simulink model "SR25"  (R2024a)
settings: Solver=FixedStepDiscrete  StartTime=0.0  StopTime=5  FixedStep=0.01  RelTol=1e-3  EnableMultiTasking=on
PreLoadFcn:
  | try, model_open; catch, disp('Error occurred while executing model pre-load callback: model_open.m'); disp('Please assure that the MATLAB working directory is set to the model directory before opening.'); end
InitFcn:
  | try, model_open; catch, end
undefined symbols (not defined in the file or in its folder): dt, GCM, raptor_get_safe_string, raptor_xcp_function
libraries: Raptor_lib x40, Utilities x13, TireTemperature x12, simulink x5, IO x5, APPS_BSPC x4, RotorTemperature x4, FlowRate x3, Cooling x2, BMS x2, Brakes x2, StateMachine x2
(part 2 of 3)

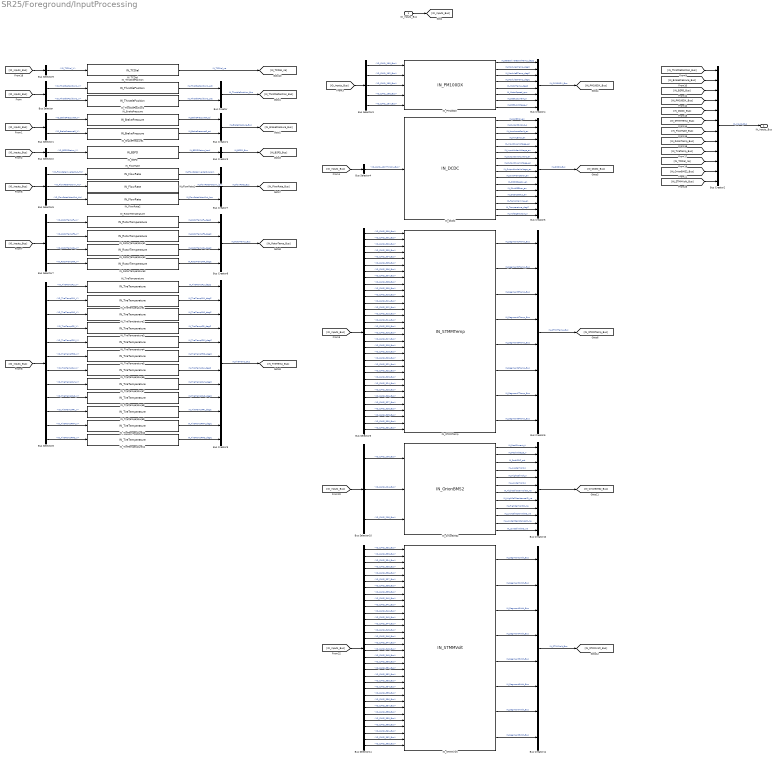
== system SR25/Foreground/InputProcessing ==
  IO_Inputs_Bus : Inport
  Bus Creator : BusCreator  Inputs=2
  Bus Creator1 : BusCreator  Inputs=2
  Bus Creator10 : BusCreator  Inputs=12
  Bus Creator11 : BusCreator  Inputs=8
  Bus Creator2 : BusCreator  Inputs=12
  Bus Creator3 : BusCreator  Inputs=1
  Bus Creator4 : BusCreator  Inputs=8
  Bus Creator5 : BusCreator  Inputs=16
  Bus Creator6 : BusCreator  Inputs=8
  Bus Creator7 : BusCreator  Inputs=3
  Bus Creator8 : BusCreator  Inputs=4
  Bus Creator9 : BusCreator  Inputs=12
  Bus Selector : BusSelector  OutputSignals=IO_AnalogInputs_Bus.IO_ThrottlePosition1_V,IO_AnalogInputs_Bus.IO_ThrottlePosition2_V
  Bus Selector1 : BusSelector  OutputSignals=IO_AnalogInputs_Bus.IO_BrakePressureF_V,IO_AnalogInputs_Bus.IO_BrakePressureR_V
  Bus Selector10 : BusSelector  OutputSignals=IO_CANInputs_Bus.IO_CAN2_Bus.IO_CAN2_BMS_Bus.IO_CAN2_200_Bus,IO_CANInputs_Bus.IO_CAN2_Bus.IO_CAN2_BMS_Bus.IO_CAN2_204_Bus,IO_CANInputs_Bus.IO_CAN2_Bus.IO_CAN2_BMS_Bus.IO_CAN2_208_Bus
  Bus Selector11 : BusSelector  OutputSignals=IO_CANInputs_Bus.IO_CAN2_Bus.IO_CAN2_STMM_Bus.IO_CAN2_STMM_Volt_Bus.IO_CAN2_332_Bus,IO_CANInputs_Bus.IO_CAN2_Bus.IO_CAN2_STMM_Bus.IO_CAN2_STMM_Volt_Bus.IO_CAN2_333_Bus,IO_CANInputs_Bus.IO_CAN2_Bus.IO_CAN2_STMM_Bus.IO_CAN2_STMM_Volt_Bus.IO_CAN2_334_Bus,IO_CANInputs_Bus.IO_CAN2_Bus.IO_CAN2_STMM_Bus.IO_CAN2_STMM_Volt_Bus.IO_CAN2_335_Bus,IO_CANInputs_Bus.IO_CAN2_Bus.IO_CAN2_STMM_Bus.IO_CAN2_STMM_Volt_Bus.IO_CAN2_336_Bus,IO_CANInputs_Bus.IO_CAN2_Bus.IO_CAN2_STMM_Bus.IO_CAN2_STMM_Volt_Bus.IO_CAN2_337_Bus,IO_CANInputs_Bus.IO_CAN2_Bus.IO_CAN2_STMM_Bus.IO_CAN2_STMM_Volt_Bus.IO_CAN2_338_Bus,IO_CANInputs_Bus.IO_CAN2_Bus.IO_CAN2_STMM_Bus.IO_CAN2_STMM_Volt_Bus.IO_CAN2_339_Bus,IO_CANInputs_Bus.IO_CAN2_Bus.IO_CAN2_STMM_Bus.IO_CAN2_STMM_Volt_Bus.IO_CAN2_340_Bus,IO_CANInputs_Bus.IO_CAN2_Bus.IO_CAN2_STMM_Bus.IO_CAN2_STMM_Volt_Bus.IO_CAN2_341_Bus,IO_CANInputs_Bus.IO_CAN2_Bus.IO_CAN2_STMM_Bus.IO_CAN2_STMM_Volt_Bus.IO_CAN2_342_Bus,IO_CANInputs_Bus.IO_CAN2_Bus.IO_CAN2_STMM_Bus.IO_CAN2_STMM_Volt_Bus.IO_CAN2_343_Bus,IO_CANInputs_Bus.IO_CAN2_Bus.IO_CAN2_STMM_Bus.IO_CAN2_STMM_Volt_Bus.IO_CAN2_344_Bus,IO_CANInputs_Bus.IO_CAN2_Bus.IO_CAN2_STMM_Bus.IO_CAN2_STMM_Volt_Bus.IO_CAN2_345_Bus,IO_CANInputs_Bus.IO_CAN2_Bus.IO_CAN2_STMM_Bus.IO_CAN2_STMM_Volt_Bus.IO_CAN2_346_Bus,IO_CANInputs_Bus.IO_CAN2_Bus.IO_CAN2_STMM_Bus.IO_CAN2_STMM_Volt_Bus.IO_CAN2_347_Bus,IO_CANInputs_Bus.IO_CAN2_Bus.IO_CAN2_STMM_Bus.IO_CAN2_STMM_Volt_Bus.IO_CAN2_348_Bus,IO_CANInputs_Bus.IO_CAN2_Bus.IO_CAN2_STMM_Bus.IO_CAN2_STMM_Volt_Bus.IO_CAN2_349_Bus,IO_CANInputs_Bus.IO_CAN2_Bus.IO_CAN2_STMM_Bus.IO_CAN2_STMM_Volt_Bus.IO_CAN2_350_Bus,IO_CANInputs_Bus.IO_CAN2_Bus.IO_CAN2_STMM_Bus.IO_CAN2_STMM_Volt_Bus.IO_CAN2_351_Bus,IO_CANInputs_Bus.IO_CAN2_Bus.IO_CAN2_STMM_Bus.IO_CAN2_STMM_Volt_Bus.IO_CAN2_352_Bus,IO_CANInputs_Bus.IO_CAN2_Bus.IO_CAN2_STMM_Bus.IO_CAN2_STMM_Volt_Bus.IO_CAN2_353_Bus,IO_CANInputs_Bus.IO_CAN2_Bus.IO_CAN2_STMM_Bus.IO_CAN2_STMM_Volt_Bus.IO_CAN2_354_Bus,IO_CANInputs_Bus.IO_CAN2_Bus.IO_CAN2_STMM_Bus.IO_CAN2_STMM_Volt_Bus.IO_CAN2_355_Bus,IO_CANInputs_Bus.IO_CAN2_Bus.IO_CAN2_STMM_Bus.IO_CAN2_STMM_Volt_Bus.IO_CAN2_356_Bus,IO_CANInputs_Bus.IO_CAN2_Bus.IO_CAN2_STMM_Bus.IO_CAN2_STMM_Volt_Bus.IO_CAN2_357_Bus,IO_CANInputs_Bus.IO_CAN2_Bus.IO_CAN2_STMM_Bus.IO_CAN2_STMM_Volt_Bus.IO_CAN2_358_Bus,IO_CANInputs_Bus.IO_CAN2_Bus.IO_CAN2_STMM_Bus.IO_CAN2_STMM_Volt_Bus.IO_CAN2_359_Bus,IO_CANInputs_Bus.IO_CAN2_Bus.IO_CAN2_STMM_Bus.IO_CAN2_STMM_Volt_Bus.IO_CAN2_360_Bus,IO_CANInputs_Bus.IO_CAN2_Bus.IO_CAN2_STMM_Bus.IO_CAN2_STMM_Volt_Bus.IO_CAN2_361_Bus,IO_CANInputs_Bus.IO_CAN2_Bus.IO_CAN2_STMM_Bus.IO_CAN2_STMM_Volt_Bus.IO_CAN2_362_Bus,IO_CANInputs_Bus.IO_CAN2_Bus.IO_CAN2_STMM_Bus.IO_CAN2_STMM_Volt_Bus.IO_CAN2_363_Bus
  Bus Selector2 : BusSelector  OutputSignals=IO_AnalogInputs_Bus.IO_BSPDStatus_V
  Bus Selector3 : BusSelector  OutputSignals=IO_CANInputs_Bus.IO_CAN1_Bus.IO_CAN1_PM100DX_Bus.IO_CAN1_160_Bus,IO_CANInputs_Bus.IO_CAN1_Bus.IO_CAN1_PM100DX_Bus.IO_CAN1_162_Bus,IO_CANInputs_Bus.IO_CAN1_Bus.IO_CAN1_PM100DX_Bus.IO_CAN1_165_Bus,IO_CANInputs_Bus.IO_CAN1_Bus.IO_CAN1_PM100DX_Bus.IO_CAN1_166_Bus,IO_CANInputs_Bus.IO_CAN1_Bus.IO_CAN1_PM100DX_Bus.IO_CAN1_167_Bus
  Bus Selector4 : BusSelector  OutputSignals=IO_CANInputs_Bus.IO_CAN1_Bus.IO_CAN1_DCDC_Bus.IO_CAN1_402772111_Bus
  Bus Selector5 : BusSelector  OutputSignals=IO_CANInputs_Bus.IO_CAN2_Bus.IO_CAN2_STMM_Bus.IO_CAN2_STMM_Temp_Bus.IO_CAN2_300_Bus,IO_CANInputs_Bus.IO_CAN2_Bus.IO_CAN2_STMM_Bus.IO_CAN2_STMM_Temp_Bus.IO_CAN2_301_Bus,IO_CANInputs_Bus.IO_CAN2_Bus.IO_CAN2_STMM_Bus.IO_CAN2_STMM_Temp_Bus.IO_CAN2_302_Bus,IO_CANInputs_Bus.IO_CAN2_Bus.IO_CAN2_STMM_Bus.IO_CAN2_STMM_Temp_Bus.IO_CAN2_303_Bus,IO_CANInputs_Bus.IO_CAN2_Bus.IO_CAN2_STMM_Bus.IO_CAN2_STMM_Temp_Bus.IO_CAN2_304_Bus,IO_CANInputs_Bus.IO_CAN2_Bus.IO_CAN2_STMM_Bus.IO_CAN2_STMM_Temp_Bus.IO_CAN2_305_Bus,IO_CANInputs_Bus.IO_CAN2_Bus.IO_CAN2_STMM_Bus.IO_CAN2_STMM_Temp_Bus.IO_CAN2_306_Bus,IO_CANInputs_Bus.IO_CAN2_Bus.IO_CAN2_STMM_Bus.IO_CAN2_STMM_Temp_Bus.IO_CAN2_307_Bus,IO_CANInputs_Bus.IO_CAN2_Bus.IO_CAN2_STMM_Bus.IO_CAN2_STMM_Temp_Bus.IO_CAN2_308_Bus,IO_CANInputs_Bus.IO_CAN2_Bus.IO_CAN2_STMM_Bus.IO_CAN2_STMM_Temp_Bus.IO_CAN2_309_Bus,IO_CANInputs_Bus.IO_CAN2_Bus.IO_CAN2_STMM_Bus.IO_CAN2_STMM_Temp_Bus.IO_CAN2_310_Bus,IO_CANInputs_Bus.IO_CAN2_Bus.IO_CAN2_STMM_Bus.IO_CAN2_STMM_Temp_Bus.IO_CAN2_311_Bus,IO_CANInputs_Bus.IO_CAN2_Bus.IO_CAN2_STMM_Bus.IO_CAN2_STMM_Temp_Bus.IO_CAN2_312_Bus,IO_CANInputs_Bus.IO_CAN2_Bus.IO_CAN2_STMM_Bus.IO_CAN2_STMM_Temp_Bus.IO_CAN2_313_Bus,IO_CANInputs_Bus.IO_CAN2_Bus.IO_CAN2_STMM_Bus.IO_CAN2_STMM_Temp_Bus.IO_CAN2_314_Bus,IO_CANInputs_Bus.IO_CAN2_Bus.IO_CAN2_STMM_Bus.IO_CAN2_STMM_Temp_Bus.IO_CAN2_315_Bus,IO_CANInputs_Bus.IO_CAN2_Bus.IO_CAN2_STMM_Bus.IO_CAN2_STMM_Temp_Bus.IO_CAN2_316_Bus,IO_CANInputs_Bus.IO_CAN2_Bus.IO_CAN2_STMM_Bus.IO_CAN2_STMM_Temp_Bus.IO_CAN2_317_Bus,IO_CANInputs_Bus.IO_CAN2_Bus.IO_CAN2_STMM_Bus.IO_CAN2_STMM_Temp_Bus.IO_CAN2_318_Bus,IO_CANInputs_Bus.IO_CAN2_Bus.IO_CAN2_STMM_Bus.IO_CAN2_STMM_Temp_Bus.IO_CAN2_319_Bus,IO_CANInputs_Bus.IO_CAN2_Bus.IO_CAN2_STMM_Bus.IO_CAN2_STMM_Temp_Bus.IO_CAN2_320_Bus,IO_CANInputs_Bus.IO_CAN2_Bus.IO_CAN2_STMM_Bus.IO_CAN2_STMM_Temp_Bus.IO_CAN2_321_Bus,IO_CANInputs_Bus.IO_CAN2_Bus.IO_CAN2_STMM_Bus.IO_CAN2_STMM_Temp_Bus.IO_CAN2_322_Bus,IO_CANInputs_Bus.IO_CAN2_Bus.IO_CAN2_STMM_Bus.IO_CAN2_STMM_Temp_Bus.IO_CAN2_323_Bus,IO_CANInputs_Bus.IO_CAN2_Bus.IO_CAN2_STMM_Bus.IO_CAN2_STMM_Temp_Bus.IO_CAN2_324_Bus,IO_CANInputs_Bus.IO_CAN2_Bus.IO_CAN2_STMM_Bus.IO_CAN2_STMM_Temp_Bus.IO_CAN2_325_Bus,IO_CANInputs_Bus.IO_CAN2_Bus.IO_CAN2_STMM_Bus.IO_CAN2_STMM_Temp_Bus.IO_CAN2_326_Bus,IO_CANInputs_Bus.IO_CAN2_Bus.IO_CAN2_STMM_Bus.IO_CAN2_STMM_Temp_Bus.IO_CAN2_327_Bus,IO_CANInputs_Bus.IO_CAN2_Bus.IO_CAN2_STMM_Bus.IO_CAN2_STMM_Temp_Bus.IO_CAN2_328_Bus,IO_CANInputs_Bus.IO_CAN2_Bus.IO_CAN2_STMM_Bus.IO_CAN2_STMM_Temp_Bus.IO_CAN2_329_Bus,IO_CANInputs_Bus.IO_CAN2_Bus.IO_CAN2_STMM_Bus.IO_CAN2_STMM_Temp_Bus.IO_CAN2_330_Bus,IO_CANInputs_Bus.IO_CAN2_Bus.IO_CAN2_STMM_Bus.IO_CAN2_STMM_Temp_Bus.IO_CAN2_331_Bus
  Bus Selector6 : BusSelector  OutputSignals=IO_DigitalInputs_Bus.IO_FlowRateInverterOut_Hz,IO_DigitalInputs_Bus.IO_FlowRateMotorIn_Hz,IO_DigitalInputs_Bus.IO_FlowRateMotorOut_Hz
  Bus Selector7 : BusSelector  OutputSignals=IO_AnalogInputs_Bus.IO_RotorTempFL_V,IO_AnalogInputs_Bus.IO_RotorTempFR_V,IO_AnalogInputs_Bus.IO_RotorTempRL_V,IO_AnalogInputs_Bus.IO_RotorTempRR_V
  Bus Selector8 : BusSelector  OutputSignals=IO_AnalogInputs_Bus.IO_TireTempFLI_V,IO_AnalogInputs_Bus.IO_TireTempFLM_V,IO_AnalogInputs_Bus.IO_TireTempFLO_V,IO_AnalogInputs_Bus.IO_TireTempFRI_V,IO_AnalogInputs_Bus.IO_TireTempFRM_V,IO_AnalogInputs_Bus.IO_TireTempFRO_V,IO_AnalogInputs_Bus.IO_TireTempRLI_V,IO_AnalogInputs_Bus.IO_TireTempRLM_V,IO_AnalogInputs_Bus.IO_TireTempRLO_V,IO_AnalogInputs_Bus.IO_TireTempRRI_V,IO_AnalogInputs_Bus.IO_TireTempRRM_V,IO_AnalogInputs_Bus.IO_TireTempRRO_V
  Bus Selector9 : BusSelector  OutputSignals=IO_AnalogInputs_Bus.IO_TCDial_V
  IN_BSPD : BSPD/IN_BSPD  pos='Status'
  IN_BrakePressure : BrakePressure/IN_BrakePressure  pos='F'
  IN_BrakePressure1 : BrakePressure/IN_BrakePressure  pos='R'
  IN_DCDC : DCDC/IN_DCDC  SystemSampleTime=-1  VariantActivationTime=update diagram  AllowFlexibleInterface=on  Latency=0  AutoFrameSizeCalculation=off
  IN_FlowRate : FlowRate/IN_FlowRate  pos='InverterOut'
  IN_FlowRate1 : FlowRate/IN_FlowRate  pos='MotorIn'
  IN_FlowRate2 : FlowRate/IN_FlowRate  pos='MotorOut'
  IN_OrionBMS2 : OrionBMS2/IN_OrionBMS2  SystemSampleTime=-1  VariantActivationTime=update diagram  AllowFlexibleInterface=on  Latency=0  AutoFrameSizeCalculation=off
  IN_PM100DX : PM100DX/IN_PM100DX  SystemSampleTime=-1  VariantActivationTime=update diagram  AllowFlexibleInterface=on  Latency=0  AutoFrameSizeCalculation=off
  IN_RotorTemperature : RotorTemperature/IN_RotorTemperature  pos='FL'
  IN_RotorTemperature1 : RotorTemperature/IN_RotorTemperature  pos='FR'
  IN_RotorTemperature2 : RotorTemperature/IN_RotorTemperature  pos='RL'
  IN_RotorTemperature3 : RotorTemperature/IN_RotorTemperature  pos='RR'
  IN_STMMTemp : STMM/IN_STMMTemp  SystemSampleTime=-1  VariantActivationTime=update diagram  AllowFlexibleInterface=on  Latency=0  AutoFrameSizeCalculation=off
  IN_STMMVolt : STMM/IN_STMMVolt  SystemSampleTime=-1  VariantActivationTime=update diagram  AllowFlexibleInterface=on  Latency=0  AutoFrameSizeCalculation=off
  IN_TCDial : TCDial/IN_TCDial  pos=''
  IN_ThrottlePosition : ThrottlePosition/IN_ThrottlePosition  pos='1'
  IN_ThrottlePosition1 : ThrottlePosition/IN_ThrottlePosition  pos='2'
  IN_TireTemperature : TireTemperature/IN_TireTemperature  pos='FLI'
  IN_TireTemperature1 : TireTemperature/IN_TireTemperature  pos='FLM'
  IN_TireTemperature10 : TireTemperature/IN_TireTemperature  pos='RRM'
  IN_TireTemperature11 : TireTemperature/IN_TireTemperature  pos='RRO'
  IN_TireTemperature2 : TireTemperature/IN_TireTemperature  pos='FLO'
  IN_TireTemperature3 : TireTemperature/IN_TireTemperature  pos='FRI'
  IN_TireTemperature4 : TireTemperature/IN_TireTemperature  pos='FRM'
  IN_TireTemperature5 : TireTemperature/IN_TireTemperature  pos='FRO'
  IN_TireTemperature6 : TireTemperature/IN_TireTemperature  pos='RLI'
  IN_TireTemperature7 : TireTemperature/IN_TireTemperature  pos='RLM'
  IN_TireTemperature8 : TireTemperature/IN_TireTemperature  pos='RLO'
  IN_TireTemperature9 : TireTemperature/IN_TireTemperature  pos='RRI'
  IN_Inputs_Bus : Outport
  wires:
  Bus Selector/1 -> IN_ThrottlePosition/1  "<IO_ThrottlePosition1_V>"
  Bus Selector/2 -> IN_ThrottlePosition1/1  "<IO_ThrottlePosition2_V>"
  IN_ThrottlePosition/1 -> Bus Creator/1  "IN_ThrottlePosition1_pct"
  IN_ThrottlePosition1/1 -> Bus Creator/2  "IN_ThrottlePosition2_pct"
  Bus Creator/1 -> [IN_ThrottlePosition_Bus]  "IN_ThrottlePosition_Bus"
  Bus Selector1/1 -> IN_BrakePressure/1  "<IO_BrakePressureF_V>"
  Bus Selector1/2 -> IN_BrakePressure1/1  "<IO_BrakePressureR_V>"
  IN_BrakePressure/1 -> Bus Creator1/1  "IN_BrakePressureF_psi"
  IN_BrakePressure1/1 -> Bus Creator1/2  "IN_BrakePressureR_psi"
  Bus Creator1/1 -> [IN_BrakePressure_Bus]  "IN_BrakePressure_Bus"
  Bus Creator2/1 -> IN_Inputs_Bus/1  "IN_Inputs_Bus"
  Bus Selector2/1 -> IN_BSPD/1  "<IO_BSPDStatus_V>"
  IN_BSPD/1 -> Bus Creator3/1  "IN_BSPDStatus_bool"
  Bus Creator3/1 -> [IN_BSPD_Bus]  "IN_BSPD_Bus"
  Bus Selector3/1 -> IN_PM100DX/1  "<IO_CAN1_160_Bus>"
  Bus Selector3/2 -> IN_PM100DX/2  "<IO_CAN1_162_Bus>"
  Bus Selector3/5 -> IN_PM100DX/5  "<IO_CAN1_167_Bus>"
  IN_PM100DX/1 -> Bus Creator4/1  "IN_GateDriverBoardTemp_degC"
  IN_PM100DX/2 -> Bus Creator4/2  "IN_ModuleATemp_degC"
  IN_PM100DX/3 -> Bus Creator4/3  "IN_ModuleBTemp_degC"
  IN_PM100DX/4 -> Bus Creator4/4  "IN_ModuleCTemp_degC"
  IN_PM100DX/5 -> Bus Creator4/5  "IN_MotorTemp_degC"
  IN_PM100DX/7 -> Bus Creator4/7  "IN_DCBusCurrent_A"
  Bus Creator4/1 -> [IN_PM100DX_Bus]  "IN_PM100DX_Bus"
  Bus Selector4/1 -> IN_DCDC/1  "<IO_CAN1_402772111_Bus>"
  IN_DCDC/1 -> Bus Creator5/1  "IN_CANError_en"
  IN_DCDC/2 -> Bus Creator5/2  "IN_CurrentOutput_A"
  IN_DCDC/3 -> Bus Creator5/3  "IN_HardwareFault_en"
  IN_DCDC/4 -> Bus Creator5/4  "IN_HVILError_en"
  IN_DCDC/5 -> Bus Creator5/5  "IN_InputOverVoltage_en"
  IN_DCDC/6 -> Bus Creator5/6  "IN_InputUnderVoltage_en"
  IN_DCDC/7 -> Bus Creator5/7  "IN_OutputOverCurrent_en"
  IN_DCDC/8 -> Bus Creator5/8  "IN_OutputOverVoltage_en"
  IN_DCDC/9 -> Bus Creator5/9  "IN_OutputUnderVoltage_en"
  IN_DCDC/10 -> Bus Creator5/10  "IN_OverTempError_en"
  IN_DCDC/11 -> Bus Creator5/11  "IN_DCDCReady_en"
  IN_DCDC/12 -> Bus Creator5/12  "IN_ShutOffError_en"
  IN_DCDC/13 -> Bus Creator5/13  "IN_DCDCStatus_en"
  IN_DCDC/14 -> Bus Creator5/14  "IN_TempWarning_en"
  IN_DCDC/15 -> Bus Creator5/15  "IN_Temperature_degC"
  IN_DCDC/16 -> Bus Creator5/16  "IN_VoltageOutput_V"
  Bus Creator5/1 -> [IN_DCDC_Bus]  "IN_DCDC_Bus"
  Bus Selector5/1 -> IN_STMMTemp/1  "<IO_CAN2_300_Bus>"
  Bus Selector5/2 -> IN_STMMTemp/2  "<IO_CAN2_301_Bus>"
  Bus Selector5/3 -> IN_STMMTemp/3  "<IO_CAN2_302_Bus>"
  Bus Selector5/4 -> IN_STMMTemp/4  "<IO_CAN2_303_Bus>"
  Bus Selector5/5 -> IN_STMMTemp/5  "<IO_CAN2_304_Bus>"
  Bus Selector5/6 -> IN_STMMTemp/6  "<IO_CAN2_305_Bus>"
  Bus Selector5/7 -> IN_STMMTemp/7  "<IO_CAN2_306_Bus>"
  Bus Selector5/8 -> IN_STMMTemp/8  "<IO_CAN2_307_Bus>"
  Bus Selector5/9 -> IN_STMMTemp/9  "<IO_CAN2_308_Bus>"
  Bus Selector5/10 -> IN_STMMTemp/10  "<IO_CAN2_309_Bus>"
  Bus Selector5/11 -> IN_STMMTemp/11  "<IO_CAN2_310_Bus>"
  Bus Selector5/12 -> IN_STMMTemp/12  "<IO_CAN2_311_Bus>"
  Bus Selector5/13 -> IN_STMMTemp/13  "<IO_CAN2_312_Bus>"
  Bus Selector5/14 -> IN_STMMTemp/14  "<IO_CAN2_313_Bus>"
  Bus Selector5/15 -> IN_STMMTemp/15  "<IO_CAN2_314_Bus>"
  Bus Selector5/16 -> IN_STMMTemp/16  "<IO_CAN2_315_Bus>"
  Bus Selector5/17 -> IN_STMMTemp/17  "<IO_CAN2_316_Bus>"
  Bus Selector5/18 -> IN_STMMTemp/18  "<IO_CAN2_317_Bus>"
  Bus Selector5/19 -> IN_STMMTemp/19  "<IO_CAN2_318_Bus>"
  Bus Selector5/20 -> IN_STMMTemp/20  "<IO_CAN2_319_Bus>"
  Bus Selector5/21 -> IN_STMMTemp/21  "<IO_CAN2_320_Bus>"
  Bus Selector5/22 -> IN_STMMTemp/22  "<IO_CAN2_321_Bus>"
  Bus Selector5/23 -> IN_STMMTemp/23  "<IO_CAN2_322_Bus>"
  Bus Selector5/24 -> IN_STMMTemp/24  "<IO_CAN2_323_Bus>"
  Bus Selector5/25 -> IN_STMMTemp/25  "<IO_CAN2_324_Bus>"
  Bus Selector5/26 -> IN_STMMTemp/26  "<IO_CAN2_325_Bus>"
  Bus Selector5/27 -> IN_STMMTemp/27  "<IO_CAN2_326_Bus>"
  Bus Selector5/28 -> IN_STMMTemp/28  "<IO_CAN2_327_Bus>"
  Bus Selector5/29 -> IN_STMMTemp/29  "<IO_CAN2_328_Bus>"
  Bus Selector5/30 -> IN_STMMTemp/30  "<IO_CAN2_329_Bus>"
  Bus Selector5/31 -> IN_STMMTemp/31  "<IO_CAN2_330_Bus>"
  Bus Selector5/32 -> IN_STMMTemp/32  "<IO_CAN2_331_Bus>"
  IN_STMMTemp/1 -> Bus Creator6/1  "IN_Segment1Temp_Bus"
  IN_STMMTemp/2 -> Bus Creator6/2  "IN_Segment2Temp_Bus"
  IN_STMMTemp/3 -> Bus Creator6/3  "IN_Segment3Temp_Bus"
  IN_STMMTemp/4 -> Bus Creator6/4  "IN_Segment4Temp_Bus"
  IN_STMMTemp/5 -> Bus Creator6/5  "IN_Segment5Temp_Bus"
  IN_STMMTemp/6 -> Bus Creator6/6  "IN_Segment6Temp_Bus"
  IN_STMMTemp/7 -> Bus Creator6/7  "IN_Segment7Temp_Bus"
  IN_STMMTemp/8 -> Bus Creator6/8  "IN_Segment8Temp_Bus"
  Bus Creator6/1 -> [IN_STMMTemp_Bus]  "IN_STMMTemp_Bus"
  Bus Selector6/1 -> IN_FlowRate/1  "<IO_FlowRateInverterOut_Hz>"
  IN_FlowRate/1 -> Bus Creator7/1  "IN_FlowRateInverterOut_lpm"
  Bus Creator7/1 -> [IN_FlowRate_Bus]  "IN_FlowRate_Bus"
  Bus Selector6/2 -> IN_FlowRate1/1  "<IO_FlowRateMotorIn_Hz>"
  Bus Selector6/3 -> IN_FlowRate2/1  "<IO_FlowRateMotorOut_Hz>"
  IN_FlowRate1/1 -> Bus Creator7/2  "IN_FlowRateMotorIn_lpm"
  IN_FlowRate2/1 -> Bus Creator7/3  "IN_FlowRateMotorOut_lpm"
  Bus Selector7/1 -> IN_RotorTemperature/1  "<IO_RotorTempFL_V>"
  Bus Selector7/2 -> IN_RotorTemperature1/1  "<IO_RotorTempFR_V>"
  Bus Selector7/3 -> IN_RotorTemperature2/1  "<IO_RotorTempRL_V>"
  Bus Selector7/4 -> IN_RotorTemperature3/1  "<IO_RotorTempRR_V>"
  IN_RotorTemperature/1 -> Bus Creator8/1  "IN_RotorTempFL_degC"
  IN_RotorTemperature1/1 -> Bus Creator8/2  "IN_RotorTempFR_degC"
  IN_RotorTemperature2/1 -> Bus Creator8/3  "IN_RotorTempRL_degC"
  IN_RotorTemperature3/1 -> Bus Creator8/4  "IN_RotorTempRR_degC"
  Bus Creator8/1 -> [IN_RotorTemp_Bus]  "IN_RotorTemp_Bus"
  Bus Selector8/1 -> IN_TireTemperature/1  "<IO_TireTempFLI_V>"
  Bus Selector8/2 -> IN_TireTemperature1/1  "<IO_TireTempFLM_V>"
  Bus Selector8/3 -> IN_TireTemperature2/1  "<IO_TireTempFLO_V>"
  Bus Selector8/4 -> IN_TireTemperature3/1  "<IO_TireTempFRI_V>"
  Bus Selector8/5 -> IN_TireTemperature4/1  "<IO_TireTempFRM_V>"
  Bus Selector8/6 -> IN_TireTemperature5/1  "<IO_TireTempFRO_V>"
  Bus Selector8/7 -> IN_TireTemperature6/1  "<IO_TireTempRLI_V>"
  Bus Selector8/8 -> IN_TireTemperature7/1  "<IO_TireTempRLM_V>"
  Bus Selector8/9 -> IN_TireTemperature8/1  "<IO_TireTempRLO_V>"
  Bus Selector8/10 -> IN_TireTemperature9/1  "<IO_TireTempRRI_V>"
  Bus Selector8/11 -> IN_TireTemperature10/1  "<IO_TireTempRRM_V>"
  Bus Selector8/12 -> IN_TireTemperature11/1  "<IO_TireTempRRO_V>"
  IN_TireTemperature/1 -> Bus Creator9/1  "IN_TireTempFLI_degC"
  IN_TireTemperature1/1 -> Bus Creator9/2  "IN_TireTempFLM_degC"
  IN_TireTemperature2/1 -> Bus Creator9/3  "IN_TireTempFLO_degC"
  IN_TireTemperature3/1 -> Bus Creator9/4  "IN_TireTempFRI_degC"
  IN_TireTemperature4/1 -> Bus Creator9/5  "IN_TireTempFRM_degC"
  IN_TireTemperature5/1 -> Bus Creator9/6  "IN_TireTempFRO_degC"
  IN_TireTemperature6/1 -> Bus Creator9/7  "IN_TireTempRLI_degC"
  IN_TireTemperature7/1 -> Bus Creator9/8  "IN_TireTempRLM_degC"
  IN_TireTemperature8/1 -> Bus Creator9/9  "IN_TireTempRLO_degC"
  IN_TireTemperature9/1 -> Bus Creator9/10  "IN_TireTempRRI_degC"
  IN_TireTemperature10/1 -> Bus Creator9/11  "IN_TireTempRRM_degC"
  IN_TireTemperature11/1 -> Bus Creator9/12  "IN_TireTempRRO_degC"
  Bus Creator9/1 -> [IN_TireTemp_Bus]  "IN_TireTemp_Bus"
  IO_Inputs_Bus/1 -> [IO_Inputs_Bus]
  [IO_Inputs_Bus] -> Bus Selector/1
  [IO_Inputs_Bus] -> Bus Selector1/1
  [IO_Inputs_Bus] -> Bus Selector2/1
  [IO_Inputs_Bus] -> Bus Selector3/1
  [IO_Inputs_Bus] -> Bus Selector4/1
  [IO_Inputs_Bus] -> Bus Selector5/1
  [IO_Inputs_Bus] -> Bus Selector6/1
  [IO_Inputs_Bus] -> Bus Selector7/1
  [IO_Inputs_Bus] -> Bus Selector8/1
  [IN_ThrottlePosition_Bus] -> Bus Creator2/1
  [IN_BrakePressure_Bus] -> Bus Creator2/2
  [IN_BSPD_Bus] -> Bus Creator2/3
  [IN_PM100DX_Bus] -> Bus Creator2/4
  [IN_DCDC_Bus] -> Bus Creator2/5
  [IN_STMMTemp_Bus] -> Bus Creator2/6
  [IN_FlowRate_Bus] -> Bus Creator2/7
  [IN_RotorTemp_Bus] -> Bus Creator2/8
  [IN_TireTemp_Bus] -> Bus Creator2/9
  [IO_Inputs_Bus] -> Bus Selector9/1
  Bus Selector9/1 -> IN_TCDial/1  "<IO_TCDial_V>"
  [IN_TCDial_na] -> Bus Creator2/10
  IN_TCDial/1 -> [IN_TCDial_na]  "IN_TCDial_na"
  [IO_Inputs_Bus] -> Bus Selector10/1
  Bus Selector10/2 -> IN_OrionBMS2/2  "<IO_CAN2_204_Bus>"
  Bus Selector10/1 -> IN_OrionBMS2/1  "<IO_CAN2_200_Bus>"
  Bus Selector10/3 -> IN_OrionBMS2/3  "<IO_CAN2_208_Bus>"
  IN_OrionBMS2/1 -> Bus Creator10/1  "IN_PackCurrent_A"
  IN_OrionBMS2/2 -> Bus Creator10/2  "IN_PackVoltage_V"
  IN_OrionBMS2/3 -> Bus Creator10/3  "IN_PackSOC_pct"
  IN_OrionBMS2/4 -> Bus Creator10/4  "IN_AvgCellVolt_V"
  IN_OrionBMS2/5 -> Bus Creator10/5  "IN_HighCellVolt_V"
  IN_OrionBMS2/6 -> Bus Creator10/6  "IN_LowCellVolt_V"
  IN_OrionBMS2/7 -> Bus Creator10/7  "IN_HighCellOpenVoltID_na"
  IN_OrionBMS2/8 -> Bus Creator10/8  "IN_HighCellResistanceID_na"
  IN_OrionBMS2/9 -> Bus Creator10/9  "IN_HighCellVoltID_na"
  IN_OrionBMS2/10 -> Bus Creator10/10  "IN_LowCellOpenVoltID_na"
  IN_OrionBMS2/11 -> Bus Creator10/11  "IN_LowCellResistanceID_na"
  IN_OrionBMS2/12 -> Bus Creator10/12  "IN_LowCellVoltID_na"
  Bus Creator10/1 -> [IN_OrionBMS2_Bus]
  [IN_OrionBMS2_Bus] -> Bus Creator2/11
  Bus Selector3/4 -> IN_PM100DX/4  "<IO_CAN1_166_Bus>"
  IN_PM100DX/8 -> Bus Creator4/8  "IN_DCBusVoltage_V"
  Bus Selector3/3 -> IN_PM100DX/3  "<IO_CAN1_165_Bus>"
  IN_PM100DX/6 -> Bus Creator4/6  "IN_MotorSpeed_rpm"
  [IO_Inputs_Bus] -> Bus Selector11/1
  Bus Selector11/1 -> IN_STMMVolt/1  "<IO_CAN2_332_Bus>"
  Bus Selector11/2 -> IN_STMMVolt/2  "<IO_CAN2_333_Bus>"
  Bus Selector11/3 -> IN_STMMVolt/3  "<IO_CAN2_334_Bus>"
  Bus Selector11/4 -> IN_STMMVolt/4  "<IO_CAN2_335_Bus>"
  Bus Selector11/5 -> IN_STMMVolt/5  "<IO_CAN2_336_Bus>"
  Bus Selector11/6 -> IN_STMMVolt/6  "<IO_CAN2_337_Bus>"
  Bus Selector11/7 -> IN_STMMVolt/7  "<IO_CAN2_338_Bus>"
  Bus Selector11/8 -> IN_STMMVolt/8  "<IO_CAN2_339_Bus>"
  Bus Selector11/9 -> IN_STMMVolt/9  "<IO_CAN2_340_Bus>"
  Bus Selector11/10 -> IN_STMMVolt/10  "<IO_CAN2_341_Bus>"
  Bus Selector11/11 -> IN_STMMVolt/11  "<IO_CAN2_342_Bus>"
  Bus Selector11/12 -> IN_STMMVolt/12  "<IO_CAN2_343_Bus>"
  Bus Selector11/13 -> IN_STMMVolt/13  "<IO_CAN2_344_Bus>"
  Bus Selector11/14 -> IN_STMMVolt/14  "<IO_CAN2_345_Bus>"
  Bus Selector11/15 -> IN_STMMVolt/15  "<IO_CAN2_346_Bus>"
  Bus Selector11/16 -> IN_STMMVolt/16  "<IO_CAN2_347_Bus>"
  Bus Selector11/17 -> IN_STMMVolt/17  "<IO_CAN2_348_Bus>"
  Bus Selector11/18 -> IN_STMMVolt/18  "<IO_CAN2_349_Bus>"
  Bus Selector11/19 -> IN_STMMVolt/19  "<IO_CAN2_350_Bus>"
  Bus Selector11/20 -> IN_STMMVolt/20  "<IO_CAN2_351_Bus>"
  Bus Selector11/21 -> IN_STMMVolt/21  "<IO_CAN2_352_Bus>"
  Bus Selector11/22 -> IN_STMMVolt/22  "<IO_CAN2_353_Bus>"
  Bus Selector11/23 -> IN_STMMVolt/23  "<IO_CAN2_354_Bus>"
  Bus Selector11/24 -> IN_STMMVolt/24  "<IO_CAN2_355_Bus>"
  Bus Selector11/25 -> IN_STMMVolt/25  "<IO_CAN2_356_Bus>"
  Bus Selector11/26 -> IN_STMMVolt/26  "<IO_CAN2_357_Bus>"
  Bus Selector11/27 -> IN_STMMVolt/27  "<IO_CAN2_358_Bus>"
  Bus Selector11/28 -> IN_STMMVolt/28  "<IO_CAN2_359_Bus>"
  Bus Selector11/29 -> IN_STMMVolt/29  "<IO_CAN2_360_Bus>"
  Bus Selector11/30 -> IN_STMMVolt/30  "<IO_CAN2_361_Bus>"
  Bus Selector11/31 -> IN_STMMVolt/31  "<IO_CAN2_362_Bus>"
  Bus Selector11/32 -> IN_STMMVolt/32  "<IO_CAN2_363_Bus>"
  IN_STMMVolt/1 -> Bus Creator11/1  "IN_Segment1Volt_Bus"
  IN_STMMVolt/2 -> Bus Creator11/2  "IN_Segment2Volt_Bus"
  IN_STMMVolt/3 -> Bus Creator11/3  "IN_Segment3Volt_Bus"
  IN_STMMVolt/4 -> Bus Creator11/4  "IN_Segment4Volt_Bus"
  IN_STMMVolt/5 -> Bus Creator11/5  "IN_Segment5Volt_Bus"
  IN_STMMVolt/6 -> Bus Creator11/6  "IN_Segment6Volt_Bus"
  IN_STMMVolt/8 -> Bus Creator11/8  "IN_Segment8Volt_Bus"
  IN_STMMVolt/7 -> Bus Creator11/7  "IN_Segment7Volt_Bus"
  Bus Creator11/1 -> [IN_STMMVolt_Bus]  "IN_STMMVolt_Bus"
  [IN_STMMVolt_Bus] -> Bus Creator2/12

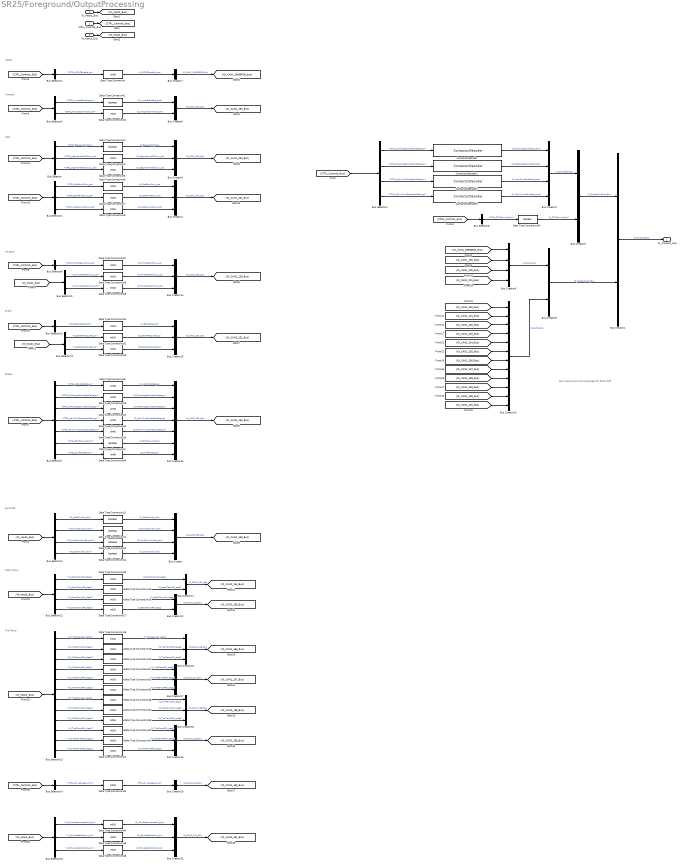
== system SR25/Foreground/OutputProcessing ==
  note: Tire Temp
  note: Rotor Temp
  note: PDM
  note: Inverter
  note: DCDC
  note: Switches
  note: Brake
  note: Throttle
  note: States
  note: also make some CAN messages for fault stuff
  IO_Inputs_Bus : Inport
  CTRL_Controls_Bus : Inport  Port=2
  IN_Inputs_Bus : Inport  Port=3
  Bus Creator : BusCreator  Inputs=4
  Bus Creator{1,5..6,8,11..12} (6 alike) : BusCreator  Inputs=2
  Bus Creator10 : BusCreator  Inputs=12
  Bus Creator13 : BusCreator  Inputs=7
  Bus Creator{3..4,14..19,21} (9 alike) : BusCreator  Inputs=3
  Bus Creator2 : BusCreator  Inputs=4
  Bus Creator20 : BusCreator  Inputs=1
  Bus Creator7 : BusCreator  Inputs=1
  Bus Creator9 : BusCreator  Inputs=4
  Bus Selector : BusSelector  OutputSignals=CTRL_BrakeLight_bool,CTRL_SegmentHalf1Duty_pct,CTRL_SegmentHalf2Duty_pct
  Bus Selector1 : BusSelector  OutputSignals=CTRL_DischargeContactorState_en,CTRL_PrechargeContactorState_en,CTRL_MainPlusContactorState_en,CTRL_MainMinusContactorState_en
  Bus Selector10 : BusSelector  OutputSignals=CTRL_BrakeBias_pct
  Bus Selector11 : BusSelector  OutputSignals=IN_BrakePressure_Bus.IN_BrakePressureF_psi,IN_BrakePressure_Bus.IN_BrakePressureR_psi
  Bus Selector12 : BusSelector  OutputSignals=IN_RotorTemp_Bus.IN_RotorTempFL_degC,IN_RotorTemp_Bus.IN_RotorTempFR_degC,IN_RotorTemp_Bus.IN_RotorTempRL_degC,IN_RotorTemp_Bus.IN_RotorTempRR_degC
  Bus Selector13 : BusSelector  OutputSignals=IN_TireTemp_Bus.IN_TireTempFLI_degC,IN_TireTemp_Bus.IN_TireTempFLM_degC,IN_TireTemp_Bus.IN_TireTempFLO_degC,IN_TireTemp_Bus.IN_TireTempFRI_degC,IN_TireTemp_Bus.IN_TireTempFRM_degC,IN_TireTemp_Bus.IN_TireTempFRO_degC,IN_TireTemp_Bus.IN_TireTempRLI_degC,IN_TireTemp_Bus.IN_TireTempRLM_degC,IN_TireTemp_Bus.IN_TireTempRLO_degC,IN_TireTemp_Bus.IN_TireTempRRI_degC,IN_TireTemp_Bus.IN_TireTempRRM_degC,IN_TireTemp_Bus.IN_TireTempRRO_degC
  Bus Selector14 : BusSelector  OutputSignals=CTRL_DriveSpeed_mph
  Bus Selector15 : BusSelector  OutputSignals=IN_FlowRate_Bus.IN_FlowRateInverterOut_lpm,IN_FlowRate_Bus.IN_FlowRateMotorIn_lpm,IN_FlowRate_Bus.IN_FlowRateMotorOut_lpm
  Bus Selector2 : BusSelector  OutputSignals=CTRL_RadFanLDuty_pct,CTRL_RadFanRDuty_pct,CTRL_WaterPumpDuty_pct
  Bus Selector3 : BusSelector  OutputSignals=IO_DigitalInputs_Bus.IO_StartSwitch_bool,IO_DigitalInputs_Bus.IO_PwrUpSwitch_bool,IO_DigitalInputs_Bus.IO_PwrDownSwitch_bool,IO_DigitalInputs_Bus.IO_CoolSwitch_bool
  Bus Selector4 : BusSelector  OutputSignals=CTRL_DCDCEnable_en
  Bus Selector5 : BusSelector  OutputSignals=CTRL_InverterEnable_en,CTRL_TorqueCommand_Nm
  Bus Selector6 : BusSelector  OutputSignals=CTRL_RTMSound_bool
  Bus Selector7 : BusSelector  OutputSignals=CTRL_VehicleState_en,CTRL_DischargeContactorState_en,CTRL_PrechargeContactorState_en,CTRL_MainPlusContactorState_en,CTRL_MainMinusContactorState_en,CTRL_RTMSound_bool,CTRL_ShifterState_en
  Bus Selector8 : BusSelector  OutputSignals=CTRL_ThrottlePosition_pct
  Bus Selector9 : BusSelector  OutputSignals=IN_ThrottlePosition_Bus.IN_ThrottlePosition1_pct,IN_ThrottlePosition_Bus.IN_ThrottlePosition2_pct
  ContactorDecoder : Utilities/ContactorDecoder  sigName='IO_DischargeContactor_bool'  contactorType=NC
  ContactorDecoder1 : Utilities/ContactorDecoder  sigName='IO_PrechargeContactor_bool'  contactorType=NO
  ContactorDecoder2 : Utilities/ContactorDecoder  sigName='IO_MainPlusContactor_bool'  contactorType=NO
  ContactorDecoder3 : Utilities/ContactorDecoder  sigName='IO_MainMinusContactor_bool'  contactorType=NO
  Data Type Conversion{,8,23..26,43} (7 alike) : DataTypeConversion  OutDataTypeStr=uint8  SaturateOnIntegerOverflow=off  RndMeth=Floor
  Data Type Conversion{1..3,11..14,34} (8 alike) : DataTypeConversion  OutDataTypeStr=boolean  SaturateOnIntegerOverflow=off  RndMeth=Floor
  Data Type Conversion{4..7,9..10,15..22,27..33,35..42,44..46} (32 alike) : DataTypeConversion  OutDataTypeStr=int16  SaturateOnIntegerOverflow=off  RndMeth=Floor
  IO_Outputs_Bus : Outport
  wires:
  Bus Creator1/1 -> IO_Outputs_Bus/1  "IO_Outputs_Bus"
  Bus Selector1/1 -> ContactorDecoder/1  "<CTRL_DischargeContactorState_en>"
  Bus Selector1/2 -> ContactorDecoder1/1  "<CTRL_PrechargeContactorState_en>"
  Bus Selector1/3 -> ContactorDecoder2/1  "<CTRL_MainPlusContactorState_en>"
  Bus Selector1/4 -> ContactorDecoder3/1  "<CTRL_MainMinusContactorState_en>"
  Bus Creator2/1 -> Bus Creator5/1  "IO_Contactor_Bus"
  Bus Creator5/1 -> Bus Creator1/1  "IO_DigitalOutputs_Bus"
  Bus Creator6/1 -> Bus Creator1/2  "IO_CANOutputs_Bus"
  ContactorDecoder/1 -> Bus Creator2/1  "IO_DischargeContactor_bool"
  ContactorDecoder1/1 -> Bus Creator2/2  "IO_PrechargeContactor_bool"
  ContactorDecoder2/1 -> Bus Creator2/3  "IO_MainPlusContactor_bool"
  ContactorDecoder3/1 -> Bus Creator2/4  "IO_MainMinusContactor_bool"
  Bus Creator7/1 -> [IO_CAN1_18008FD0_Bus]  "IO_CAN1_18008FD0_Bus"
  Bus Creator8/1 -> [IO_CAN1_192_Bus]  "IO_CAN1_192_Bus"
  Bus Creator9/1 -> Bus Creator6/1  "IO_CAN1_Bus"
  Bus Creator10/1 -> Bus Creator6/2  "IO_CAN2_Bus"
  Bus Selector4/1 -> Data Type Conversion/1  "<CTRL_DCDCEnable_en>"
  Bus Selector5/1 -> Data Type Conversion1/1  "<CTRL_InverterEnable_en>"
  Bus Selector5/2 -> Data Type Conversion22/1  "<CTRL_TorqueCommand_Nm>"
  Data Type Conversion/1 -> Bus Creator7/1  "IO_DCDCEnable_bool"
  Data Type Conversion1/1 -> Bus Creator8/1  "IO_InverterEnable_bool"
  Bus Selector6/1 -> Data Type Conversion34/1  "<CTRL_RTMSound_bool>"
  Data Type Conversion22/1 -> Bus Creator8/2  "IO_TorqueCommand_Nm"
  IO_Inputs_Bus/1 -> [IO_Inputs_Bus]
  CTRL_Controls_Bus/1 -> [CTRL_Controls_Bus]
  IN_Inputs_Bus/1 -> [IN_Inputs_Bus]
  [CTRL_Controls_Bus] -> Bus Selector1/1
  [CTRL_Controls_Bus] -> Bus Selector6/1
  [CTRL_Controls_Bus] -> Bus Selector4/1
  [CTRL_Controls_Bus] -> Bus Selector5/1
  [CTRL_Controls_Bus] -> Bus Selector7/1
  Bus Selector7/1 -> Data Type Conversion8/1  "<CTRL_VehicleState_en>"
  Bus Selector7/2 -> Data Type Conversion23/1  "<CTRL_DischargeContactorState_en>"
  Bus Selector7/3 -> Data Type Conversion24/1  "<CTRL_PrechargeContactorState_en>"
  Bus Selector7/4 -> Data Type Conversion25/1  "<CTRL_MainPlusContactorState_en>"
  Bus Selector7/5 -> Data Type Conversion26/1  "<CTRL_MainMinusContactorState_en>"
  Data Type Conversion8/1 -> Bus Creator13/1  "IO_VehicleState_en"
  Data Type Conversion23/1 -> Bus Creator13/2  "IO_DischargeContactorState_en"
  Data Type Conversion24/1 -> Bus Creator13/3  "IO_PrechargeContactorState_en"
  Data Type Conversion25/1 -> Bus Creator13/4  "IO_MainPlusContactorState_en"
  Data Type Conversion26/1 -> Bus Creator13/5  "IO_MainMinusContactorState_en"
  Bus Creator13/1 -> [IO_CAN2_152_Bus]  "IO_CAN2_152_Bus"
  Bus Creator3/1 -> [IO_CAN1_200_Bus]  "IO_CAN1_200_Bus"
  [CTRL_Controls_Bus] -> Bus Selector8/1
  [IN_Inputs_Bus] -> Bus Selector9/1
  Bus Selector8/1 -> Data Type Conversion27/1  "<CTRL_ThrottlePosition_pct>"
  Bus Selector9/1 -> Data Type Conversion28/1  "<IN_ThrottlePosition1_pct>"
  Bus Selector9/2 -> Data Type Conversion29/1  "<IN_ThrottlePosition2_pct>"
  Data Type Conversion27/1 -> Bus Creator14/1  "IO_ThrottlePosition_pct"
  Data Type Conversion28/1 -> Bus Creator14/2  "IO_ThrottlePosition1_pct"
  Data Type Conversion29/1 -> Bus Creator14/3  "IO_ThrottlePosition2_pct"
  Bus Creator14/1 -> [IO_CAN2_150_Bus]  "IO_CAN2_150_Bus"
  [CTRL_Controls_Bus] -> Bus Selector10/1
  [IN_Inputs_Bus] -> Bus Selector11/1
  Bus Selector10/1 -> Data Type Conversion31/1  "<CTRL_BrakeBias_pct>"
  Bus Selector11/1 -> Data Type Conversion32/1  "<IN_BrakePressureF_psi>"
  Bus Selector11/2 -> Data Type Conversion33/1  "<IN_BrakePressureR_psi>"
  Data Type Conversion31/1 -> Bus Creator15/1  "IO_BrakeBias_pct"
  Data Type Conversion32/1 -> Bus Creator15/2  "IO_BrakePressureF_psi"
  Data Type Conversion33/1 -> Bus Creator15/3  "IO_BrakePressureR_psi"
  Data Type Conversion34/1 -> Bus Creator5/2  "IO_RTMSound_bool"
  Bus Creator15/1 -> [IO_CAN2_151_Bus]  "IO_CAN2_151_Bus"
  [CTRL_Controls_Bus] -> Bus Selector/1
  Bus Selector/1 -> Data Type Conversion2/1  "<CTRL_BrakeLight_bool>"
  Data Type Conversion2/1 -> Bus Creator3/1  "IO_BrakeLight_bool"
  Data Type Conversion3/1 -> Bus Creator13/6  "IO_RTMSound_bool"
  Bus Selector7/6 -> Data Type Conversion3/1  "<CTRL_RTMSound_bool>"
  [IO_CAN1_18008FD0_Bus] -> Bus Creator9/1
  [IO_CAN1_192_Bus] -> Bus Creator9/2
  [IO_CAN1_200_Bus] -> Bus Creator9/3
  [IO_CAN2_150_Bus] -> Bus Creator10/1
  [IO_CAN2_151_Bus] -> Bus Creator10/2
  [IO_CAN2_152_Bus] -> Bus Creator10/3
  Data Type Conversion11/1 -> Bus Creator/1  "IO_StartSwitch_bool"
  Bus Selector3/3 -> Data Type Conversion13/1  "<IO_PwrDownSwitch_bool>"
  Bus Selector3/4 -> Data Type Conversion14/1  "<IO_CoolSwitch_bool>"
  Bus Selector3/1 -> Data Type Conversion11/1  "<IO_StartSwitch_bool>"
  Data Type Conversion12/1 -> Bus Creator/2  "IO_PwrUpSwitch_bool"
  Data Type Conversion14/1 -> Bus Creator/4  "IO_CoolSwitch_bool"
  Bus Selector3/2 -> Data Type Conversion12/1  "<IO_PwrUpSwitch_bool>"
  Data Type Conversion13/1 -> Bus Creator/3  "IO_PwrDownSwitch_bool"
  [IO_Inputs_Bus] -> Bus Selector3/1
  Bus Creator/1 -> [IO_CAN2_153_Bus]  "IO_CAN2_153_Bus"
  [IO_CAN2_153_Bus] -> Bus Creator10/4
  Bus Selector/2 -> Data Type Conversion4/1  "<CTRL_SegmentHalf1Duty_pct>"
  Bus Selector/3 -> Data Type Conversion5/1  "<CTRL_SegmentHalf2Duty_pct>"
  Data Type Conversion4/1 -> Bus Creator3/2  "IO_SegmentHalf1Duty_pct"
  Data Type Conversion5/1 -> Bus Creator3/3  "IO_SegmentHalf2Duty_pct"
  [CTRL_Controls_Bus] -> Bus Selector2/1
  Bus Selector2/1 -> Data Type Conversion6/1  "<CTRL_RadFanLDuty_pct>"
  Data Type Conversion6/1 -> Bus Creator4/1  "IO_RadFanLDuty_pct"
  Data Type Conversion7/1 -> Bus Creator4/2  "IO_RadFanRDuty_pct"
  Bus Selector2/2 -> Data Type Conversion7/1  "<CTRL_RadFanRDuty_pct>"
  Bus Selector2/3 -> Data Type Conversion9/1  "<CTRL_WaterPumpDuty_pct>"
  Data Type Conversion9/1 -> Bus Creator4/3  "IO_WaterPumpDuty_pct"
  Bus Creator4/1 -> [IO_CAN1_201_Bus]  "IO_CAN1_201_Bus"
  [IO_CAN1_201_Bus] -> Bus Creator9/4
  [IN_Inputs_Bus] -> Bus Selector12/1
  Bus Selector12/1 -> Data Type Conversion10/1  "<IN_RotorTempFL_degC>"
  Bus Selector12/4 -> Data Type Conversion17/1  "<IN_RotorTempRR_degC>"
  Bus Selector12/3 -> Data Type Conversion16/1  "<IN_RotorTempRL_degC>"
  Bus Selector12/2 -> Data Type Conversion15/1  "<IN_RotorTempFR_degC>"
  Data Type Conversion10/1 -> Bus Creator11/1  "IN_RotorTempFL_degC"
  Data Type Conversion15/1 -> Bus Creator11/2  "IN_RotorTempFR_degC"
  Data Type Conversion16/1 -> Bus Creator12/1  "IN_RotorTempRL_degC"
  Data Type Conversion17/1 -> Bus Creator12/2  "IN_RotorTempRR_degC"
  Bus Creator11/1 -> [IO_CAN2_154_Bus]  "IO_CAN2_154_Bus"
  Bus Creator12/1 -> [IO_CAN2_155_Bus]  "IO_CAN2_155_Bus"
  [IO_CAN2_154_Bus] -> Bus Creator10/5
  [IO_CAN2_155_Bus] -> Bus Creator10/6
  [IN_Inputs_Bus] -> Bus Selector13/1
  Bus Selector13/1 -> Data Type Conversion18/1  "<IN_TireTempFLI_degC>"
  Bus Selector13/2 -> Data Type Conversion19/1  "<IN_TireTempFLM_degC>"
  Bus Selector13/3 -> Data Type Conversion20/1  "<IN_TireTempFLO_degC>"
  Bus Selector13/4 -> Data Type Conversion21/1  "<IN_TireTempFRI_degC>"
  Bus Selector13/5 -> Data Type Conversion30/1  "<IN_TireTempFRM_degC>"
  Bus Selector13/6 -> Data Type Conversion35/1  "<IN_TireTempFRO_degC>"
  Bus Selector13/7 -> Data Type Conversion36/1  "<IN_TireTempRLI_degC>"
  Bus Selector13/8 -> Data Type Conversion37/1  "<IN_TireTempRLM_degC>"
  Bus Selector13/9 -> Data Type Conversion38/1  "<IN_TireTempRLO_degC>"
  Bus Selector13/10 -> Data Type Conversion39/1  "<IN_TireTempRRI_degC>"
  Bus Selector13/11 -> Data Type Conversion40/1  "<IN_TireTempRRM_degC>"
  Bus Selector13/12 -> Data Type Conversion41/1  "<IN_TireTempRRO_degC>"
  Data Type Conversion18/1 -> Bus Creator16/1  "IN_TireTempFLI_degC"
  Data Type Conversion19/1 -> Bus Creator16/2  "IN_TireTempFLM_degC"
  Data Type Conversion20/1 -> Bus Creator16/3  "IN_TireTempFLO_degC"
  Bus Creator16/1 -> [IO_CAN2_156_Bus]  "IO_CAN2_156_Bus"
  Data Type Conversion21/1 -> Bus Creator17/1  "IN_TireTempFRI_degC"
  Data Type Conversion30/1 -> Bus Creator17/2  "IN_TireTempFRM_degC"
  Data Type Conversion35/1 -> Bus Creator17/3  "IN_TireTempFRO_degC"
  Bus Creator17/1 -> [IO_CAN2_157_Bus]  "IO_CAN2_157_Bus"
  Data Type Conversion36/1 -> Bus Creator18/1  "IN_TireTempRLI_degC"
  Data Type Conversion37/1 -> Bus Creator18/2  "IN_TireTempRLM_degC"
  Data Type Conversion38/1 -> Bus Creator18/3  "IN_TireTempRLO_degC"
  Bus Creator18/1 -> [IO_CAN2_158_Bus]  "IO_CAN2_158_Bus"
  Data Type Conversion39/1 -> Bus Creator19/1  "IN_TireTempRRI_degC"
  Data Type Conversion40/1 -> Bus Creator19/2  "IN_TireTempRRM_degC"
  Data Type Conversion41/1 -> Bus Creator19/3  "IN_TireTempRRO_degC"
  Bus Creator19/1 -> [IO_CAN2_159_Bus]  "IO_CAN2_159_Bus"
  [IO_CAN2_156_Bus] -> Bus Creator10/7
  [IO_CAN2_157_Bus] -> Bus Creator10/8
  [IO_CAN2_158_Bus] -> Bus Creator10/9
  [IO_CAN2_159_Bus] -> Bus Creator10/10
  [CTRL_Controls_Bus] -> Bus Selector14/1
  Bus Selector14/1 -> Data Type Conversion42/1  "<CTRL_DriveSpeed_mph>"
  Data Type Conversion42/1 -> Bus Creator20/1  "CTRL_DriveSpeed_mph"
  Bus Creator20/1 -> [IO_CAN2_160_Bus]  "IO_CAN2_160_Bus"
  [IO_CAN2_160_Bus] -> Bus Creator10/11
  Bus Selector7/7 -> Data Type Conversion43/1  "<CTRL_ShifterState_en>"
  Data Type Conversion43/1 -> Bus Creator13/7  "IO_ShifterState_en"
  [IN_Inputs_Bus] -> Bus Selector15/1
  Bus Selector15/3 -> Data Type Conversion46/1  "<IN_FlowRateMotorOut_lpm>"
  Bus Selector15/2 -> Data Type Conversion45/1  "<IN_FlowRateMotorIn_lpm>"
  Bus Selector15/1 -> Data Type Conversion44/1  "<IN_FlowRateInverterOut_lpm>"
  Data Type Conversion45/1 -> Bus Creator21/2  "IO_FlowRateMotorIn_lpm"
  Data Type Conversion44/1 -> Bus Creator21/1  "IO_FlowRateInverterOut_lpm"
  Data Type Conversion46/1 -> Bus Creator21/3  "IO_FlowRateMotorOut_lpm"
  Bus Creator21/1 -> [IO_CAN2_161_Bus]  "IO_CAN2_161_Bus"
  [IO_CAN2_161_Bus] -> Bus Creator10/12

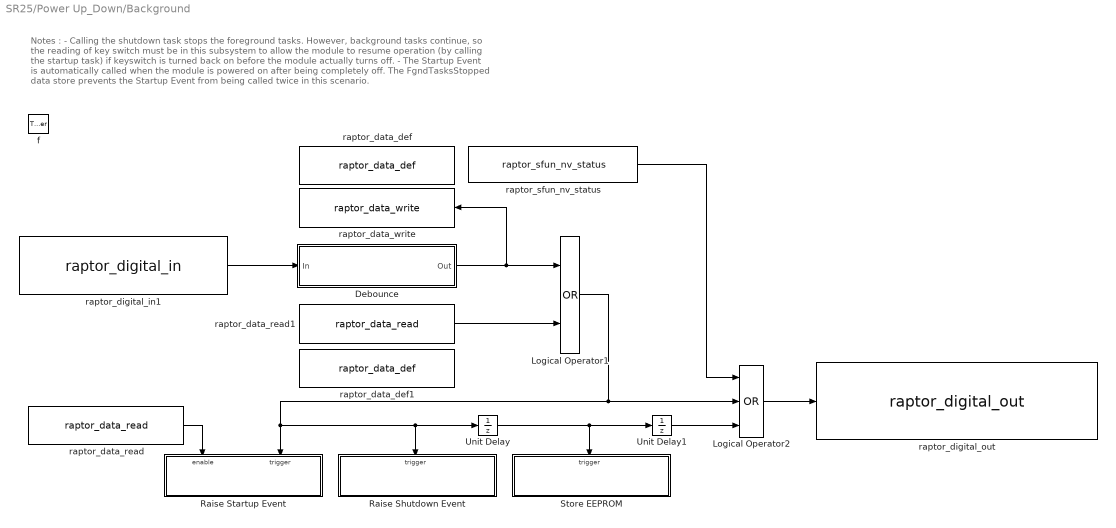
== system SR25/Power Up_Down/Background ==
  note: Notes :
      | - Calling the shutdown task stops the foreground tasks. However, background tasks continue, so the reading of key switch must be in this subsystem to allow the module
      | to resume operation (by calling the startup task) if keyswitch is turned back on before the module actually turns off.
      | - The Startup Event is automatically called when the module is powered on after being completely off. The FgndTasksStopped data store prevents the Startup Event from being called twice in this scenario.
  f : TriggerPort  TriggerType=function-call  VariantControl=Variant  ZeroCross=off
  Debounce : Subsystem
  Logical Operator1 : Logic  Operator=OR  OutDataTypeStr=boolean
  Logical Operator2 : Logic  Operator=OR  Inputs=3  OutDataTypeStr=boolean
  Raise Shutdown Event : Subsystem  TreatAsAtomicUnit=on
  Raise Startup Event : Subsystem  TreatAsAtomicUnit=on
  Store EEPROM : Subsystem  TreatAsAtomicUnit=on
  Unit Delay : UnitDelay  SampleTime=-1  HasFrameUpgradeWarning=on
  Unit Delay1 : UnitDelay  SampleTime=-1  HasFrameUpgradeWarning=on
  raptor_data_def : Raptor_lib/Data Storage/raptor_data_def  dataName='KeySw_Bgnd'  initValue=0  dataType=boolean  storage=Volatile (RAM)  calVisible=on  calType=Measurement  calDispType=Number  calEnum={'False', 'True'}  calGain=1.0  calOffset=0  calMin=-Inf  calMax=Inf  calFormat='-1'  calUnit='Bool'  calHelp='Key switch reading from background task'  calAccess=1  calFunction=group  calDispHeaders=off  calColHeaders={'Col1' 'Col2' 'Col3'}  calRowHeaders={'Row1' 'Row2' 'Row3'}
      settings: SourceProductName=Raptor
  raptor_data_def1 : Raptor_lib/Data Storage/raptor_data_def  dataName='KeepModuleOn'  initValue=0  dataType=boolean  storage=Volatile (RAM)  calVisible=on  calType=Measurement  calDispType=Number  calEnum={'False', 'True'}  calGain=1.0  calOffset=0  calMin=-Inf  calMax=Inf  calFormat='-1'  calUnit='Bool'  calHelp='Boolean indicating module to be kept on'  calAccess=1  calFunction=group  calDispHeaders=off  calColHeaders={'Col1' 'Col2' 'Col3'}  calRowHeaders={'Row1' 'Row2' 'Row3'}
      settings: SourceProductName=Raptor
  raptor_data_read : Raptor_lib/Data Storage/raptor_data_read  dataName='FgndTasksStopped'  dataShape=Scalar  idxSource=Input  idxRow=1  idxCol=1
      settings: SourceProductName=Raptor
  raptor_data_read1 : Raptor_lib/Data Storage/raptor_data_read  dataName='KeepModuleOn'  dataShape=Scalar  idxSource=Input  idxRow=1  idxCol=1
      settings: SourceProductName=Raptor
  raptor_data_write : Raptor_lib/Data Storage/raptor_data_write  dataName='KeySw_Bgnd'  dataShape=Scalar  idxSource=Input Port  idxRow=1  idxCol=1
      settings: SourceProductName=Raptor
  raptor_digital_in1 : Raptor_lib/Input & Output/raptor_digital_in  resourceValues=WAKE_INPUT1|INPUT33|INPUT34|INPUT35|INPUT36|INPUT37|INPUT38|INPUT39|INPUT40|(None)  resource=WAKE_INPUT1  pullUDValues=2.9k PD  pullUD=(None)  upperThres='RAPTOR MASK DEFAULT'  lowerThres='RAPTOR MASK DEFAULT'
      settings: SourceProductName=Raptor
  raptor_digital_out : Raptor_lib/Input & Output/raptor_digital_out  resourceValues=OUTPUT1|OUTPUT2|OUTPUT3|OUTPUT4|OUTPUT5|OUTPUT6|OUTPUT7|OUTPUT8|OUTPUT9|OUTPUT10|OUTPUT11|OUTPUT12|OUTPUT21|OUTPUT22|OUTPUT23|OUTPUT24|OUTPUT25|OUTPUT26|OUTPUT27|OUTPUT28|OUTPUT29|OUTPUT30|OUTPUT31|OUTPUT32|OUTPUT33|OUTPUT34|OUTPUT35|OUTPUT36|OUTPUT37|OUTPUT38|OUTPUT39|OUTPUT40|OUTPUT41|OUTPUT42|OUTPUT43|OUTPUT44|OUTPUT45|OUTPUT46|OUTPUT47|OUTPUT48|OUTPUT49|POWER_HOLD|(None)  resource=POWER_HOLD  driverTypeValues=(None)  driverType=(None)
      settings: SourceProductName=Raptor
  raptor_sfun_nv_status : Raptor_lib/Data Storage/raptor_sfun_nv_status  showStatus=Store In Progess
      settings: SourceProductName=Raptor
  wires:
  raptor_data_read/1 -> Raise Startup Event/Enable
  raptor_digital_in1/1 -> Debounce/1(In)
  Logical Operator2/1 -> raptor_digital_out/1
  Unit Delay/1 -> Store EEPROM/Trigger, Unit Delay1/1
  Logical Operator1/1 -> Logical Operator2/2, Raise Startup Event/Trigger, Raise Shutdown Event/Trigger, Unit Delay/1
  Unit Delay1/1 -> Logical Operator2/3
  raptor_sfun_nv_status/1 -> Logical Operator2/1
  raptor_data_read1/1 -> Logical Operator1/2
  Debounce/1(Out) -> raptor_data_write/1, Logical Operator1/1

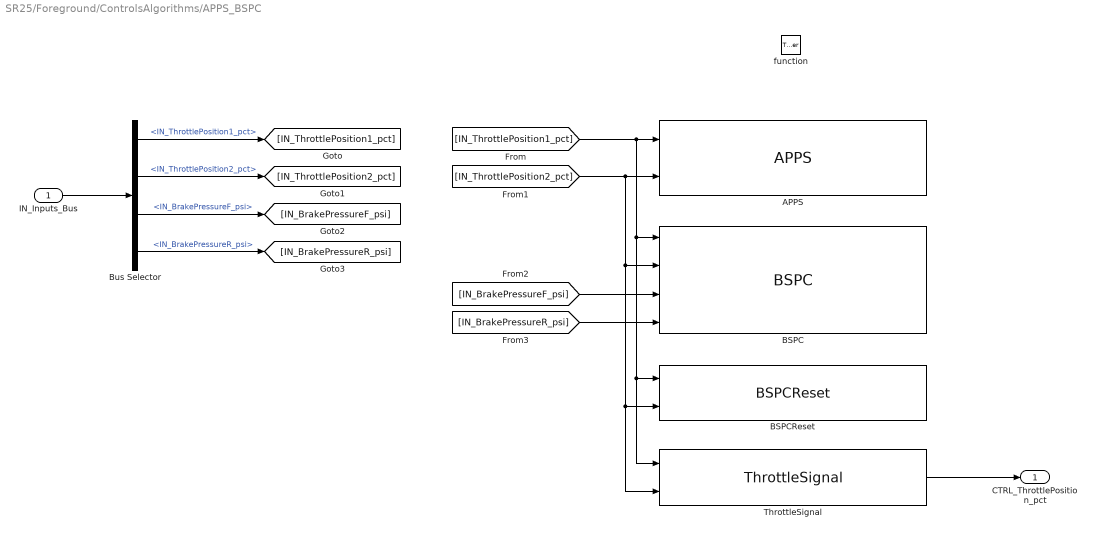
== system SR25/Foreground/ControlsAlgorithms/APPS_BSPC ==
  IN_Inputs_Bus : Inport
  function : TriggerPort  TriggerType=function-call  VariantControl=(inherit)
  APPS : APPS_BSPC/APPS  SystemSampleTime=-1  VariantActivationTime=update diagram  AllowFlexibleInterface=on  Latency=0  AutoFrameSizeCalculation=off
  BSPC : APPS_BSPC/BSPC  SystemSampleTime=-1  VariantActivationTime=update diagram  AllowFlexibleInterface=on  Latency=0  AutoFrameSizeCalculation=off
  BSPCReset : APPS_BSPC/BSPCReset  SystemSampleTime=-1  VariantActivationTime=update diagram  AllowFlexibleInterface=on  Latency=0  AutoFrameSizeCalculation=off
  Bus Selector : BusSelector  OutputSignals=IN_ThrottlePosition_Bus.IN_ThrottlePosition1_pct,IN_ThrottlePosition_Bus.IN_ThrottlePosition2_pct,IN_BrakePressure_Bus.IN_BrakePressureF_psi,IN_BrakePressure_Bus.IN_BrakePressureR_psi
  ThrottleSignal : APPS_BSPC/ThrottleSignal  SystemSampleTime=-1  VariantActivationTime=update diagram  AllowFlexibleInterface=on  Latency=0  AutoFrameSizeCalculation=off
  CTRL_ThrottlePosition_pct : Outport
  wires:
  IN_Inputs_Bus/1 -> Bus Selector/1
  Bus Selector/1 -> [IN_ThrottlePosition1_pct]  "<IN_ThrottlePosition1_pct>"
  Bus Selector/2 -> [IN_ThrottlePosition2_pct]  "<IN_ThrottlePosition2_pct>"
  Bus Selector/3 -> [IN_BrakePressureF_psi]  "<IN_BrakePressureF_psi>"
  Bus Selector/4 -> [IN_BrakePressureR_psi]  "<IN_BrakePressureR_psi>"
  [IN_ThrottlePosition1_pct] -> ThrottleSignal/1, BSPCReset/1, BSPC/1, APPS/1
  [IN_ThrottlePosition2_pct] -> ThrottleSignal/2, BSPCReset/2, BSPC/2, APPS/2
  [IN_BrakePressureF_psi] -> BSPC/3
  [IN_BrakePressureR_psi] -> BSPC/4
  ThrottleSignal/1 -> CTRL_ThrottlePosition_pct/1

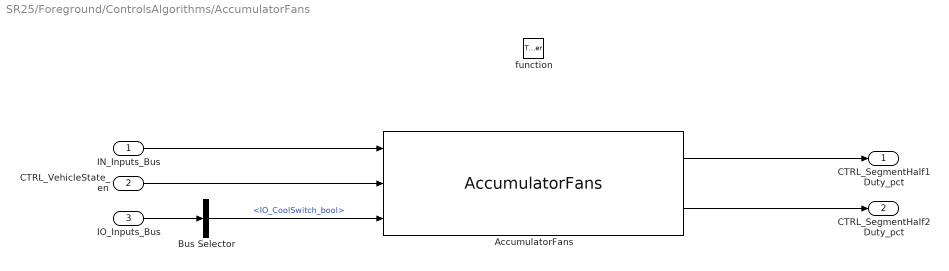
== system SR25/Foreground/ControlsAlgorithms/AccumulatorFans ==
  IN_Inputs_Bus : Inport
  CTRL_VehicleState_en : Inport  Port=2
  IO_Inputs_Bus : Inport  Port=3
  function : TriggerPort  TriggerType=function-call  VariantControl=(inherit)
  AccumulatorFans : Cooling/AccumulatorFans  SystemSampleTime=-1  VariantActivationTime=update diagram  AllowFlexibleInterface=on  Latency=0  AutoFrameSizeCalculation=off
  Bus Selector : BusSelector  OutputSignals=IO_DigitalInputs_Bus.IO_CoolSwitch_bool
  CTRL_SegmentHalf1Duty_pct : Outport
  CTRL_SegmentHalf2Duty_pct : Outport  Port=2
  wires:
  IN_Inputs_Bus/1 -> AccumulatorFans/1
  CTRL_VehicleState_en/1 -> AccumulatorFans/2
  IO_Inputs_Bus/1 -> Bus Selector/1
  Bus Selector/1 -> AccumulatorFans/3  "<IO_CoolSwitch_bool>"
  AccumulatorFans/1 -> CTRL_SegmentHalf1Duty_pct/1
  AccumulatorFans/2 -> CTRL_SegmentHalf2Duty_pct/1

== system SR25/Foreground/ControlsAlgorithms/BMS ==
  IN_Inputs_Bus : Inport
  function : TriggerPort  TriggerType=function-call  VariantControl=(inherit)
  BMSTemp : BMS/BMSTemp  SystemSampleTime=-1  VariantActivationTime=update diagram  AllowFlexibleInterface=on  Latency=0  AutoFrameSizeCalculation=off
  BMSVolt : BMS/BMSVolt  SystemSampleTime=-1  VariantActivationTime=update diagram  AllowFlexibleInterface=on  Latency=0  AutoFrameSizeCalculation=off
  Bus Selector : BusSelector  OutputSignals=IN_STMMVolt_Bus
  Bus Selector1 : BusSelector  OutputSignals=IN_STMMTemp_Bus
  wires:
  IN_Inputs_Bus/1 -> Bus Selector1/1, Bus Selector/1
  Bus Selector/1 -> BMSVolt/1  "<IN_STMMVolt_Bus>"
  Bus Selector1/1 -> BMSTemp/1  "<IN_STMMTemp_Bus>"

== system SR25/Foreground/ControlsAlgorithms/BrakeBias ==
  IN_Inputs_Bus : Inport
  function : TriggerPort  TriggerType=function-call  VariantControl=(inherit)
  BrakeBias : Brakes/BrakeBias  SystemSampleTime=-1  VariantActivationTime=update diagram  AllowFlexibleInterface=on  Latency=0  AutoFrameSizeCalculation=off
  Bus Selector : BusSelector  OutputSignals=IN_BrakePressure_Bus.IN_BrakePressureF_psi,IN_BrakePressure_Bus.IN_BrakePressureR_psi
  CTRL_BrakeBias_pct : Outport
  wires:
  IN_Inputs_Bus/1 -> Bus Selector/1
  Bus Selector/1 -> BrakeBias/1  "<IN_BrakePressureF_psi>"
  Bus Selector/2 -> BrakeBias/2  "<IN_BrakePressureR_psi>"
  BrakeBias/1 -> CTRL_BrakeBias_pct/1

== system SR25/Foreground/ControlsAlgorithms/BrakeLight ==
  IN_Inputs_Bus : Inport
  function : TriggerPort  TriggerType=function-call  VariantControl=(inherit)
  BrakeLight : Brakes/BrakeLight  SystemSampleTime=-1  VariantActivationTime=update diagram  AllowFlexibleInterface=on  Latency=0  AutoFrameSizeCalculation=off
  Bus Selector : BusSelector  OutputSignals=IN_BrakePressure_Bus.IN_BrakePressureF_psi,IN_BrakePressure_Bus.IN_BrakePressureR_psi
  CTRL_BrakeLight_bool : Outport
  wires:
  IN_Inputs_Bus/1 -> Bus Selector/1
  Bus Selector/1 -> BrakeLight/1  "<IN_BrakePressureF_psi>"
  Bus Selector/2 -> BrakeLight/2  "<IN_BrakePressureR_psi>"
  BrakeLight/1 -> CTRL_BrakeLight_bool/1

== system SR25/Foreground/ControlsAlgorithms/ClearAllFaults ==
  function : TriggerPort  TriggerType=function-call  VariantControl=(inherit)
  raptor_fault_clear : Raptor_lib/Faults/raptor_fault_clear  faultSource=All  faultName='myFault'
      settings: SourceProductName=Raptor

== system SR25/Foreground/ControlsAlgorithms/DriveSpeed ==
  IN_Inputs_Bus : Inport
  function : TriggerPort  TriggerType=function-call  VariantControl=(inherit)
  Bus Selector : BusSelector  OutputSignals=IN_PM100DX_Bus.IN_MotorSpeed_rpm
  DriveSpeed : VehicleDynamics/DriveSpeed  SystemSampleTime=-1  VariantActivationTime=update diagram  AllowFlexibleInterface=on  Latency=0  AutoFrameSizeCalculation=off
  CTRL_DriveSpeed_mph : Outport
  wires:
  IN_Inputs_Bus/1 -> Bus Selector/1
  Bus Selector/1 -> DriveSpeed/1  "<IN_MotorSpeed_rpm>"
  DriveSpeed/1 -> CTRL_DriveSpeed_mph/1

== system SR25/Foreground/ControlsAlgorithms/RTMSound ==
  CTRL_VehicleState_en : Inport
  function : TriggerPort  TriggerType=function-call  VariantControl=(inherit)
  RTMSound : StateMachine/RTMSound  SystemSampleTime=-1  VariantActivationTime=update diagram  AllowFlexibleInterface=on  Latency=0  AutoFrameSizeCalculation=off
  CTRL_RTMSound_bool : Outport
  wires:
  CTRL_VehicleState_en/1 -> RTMSound/1
  RTMSound/1 -> CTRL_RTMSound_bool/1
